simulink model "TestAgeingImpact_Intermediate_CC_Cycles"  (R2024b)
settings: Solver=FixedStepAuto  StartTime=0.0  StopTime=simTime  FixedStep=Ts  RelTol=1e-3
values from neighbouring files (symbols this model uses):
  I_ch = -OneC/Crate*A*p.L_n*p.a_s_n    [TestParallelCells.m]    (also in simu_ageing_Internediaire.m = -OneC/Crate*A_e; simu_ageing_Internediaire_3HYP.m = -OneC/Crate*A_e; simu_effet_ageing.m = -OneC/Crate)
  Ts = p.delta_t    [TestParallelCells.m]    (also in simu_ageing_Internediaire.m; simu_ageing_Internediaire_3HYP.m; simu_effet_ageing.m)
undefined symbols (not defined in the file or in its folder): p
libraries: nesl_utility x9, fl_lib x5, EHMCell_lib x2, BatteryCurrentManagement x1, spspowerguiLib x1
settings Model: Creator=lab01  LastModifiedBy=chloe

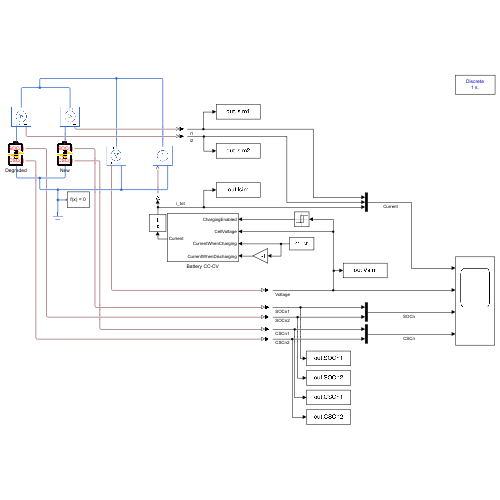
[thumbnail: Simulink's stored preview of the top-level diagram]
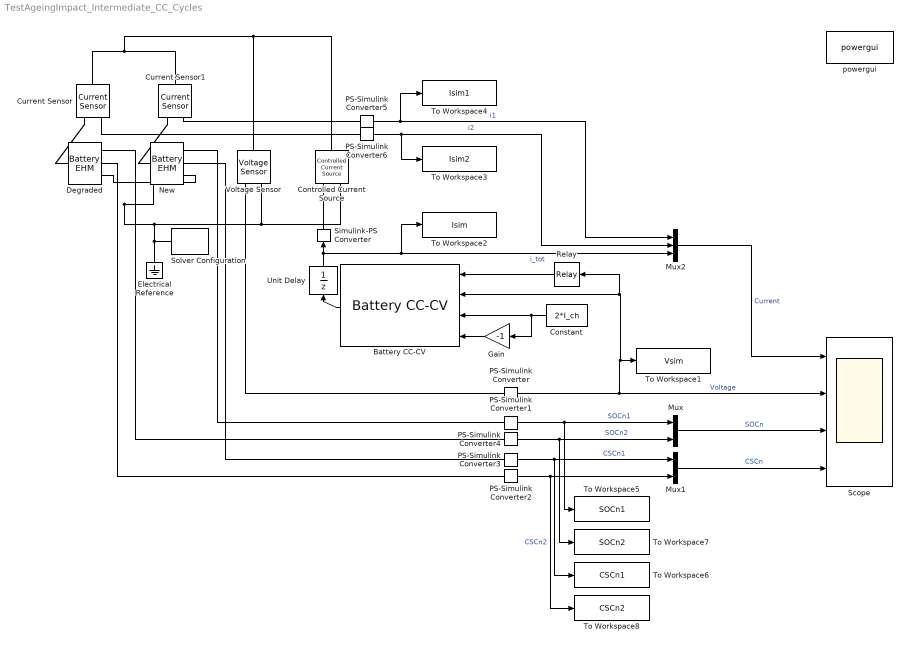
== system TestAgeingImpact_Intermediate_CC_Cycles ==
  Battery CC-CV : BatteryCurrentManagement/Battery CC-CV  MaxCellVoltage=p.volt_max  Kp=100  Ki=10  Kaw=1  Kt=1  Ts=Ts
      settings: LibrarySourceBlock=batt_sl_lib/Current Management/Battery CC-CV
  Constant : Constant  Value=2*I_ch
  Controlled Current Source : fl_lib/Electrical/Electrical Sources/Controlled Current Source
  Current Sensor : fl_lib/Electrical/Electrical Sensors/Current Sensor
  Current Sensor1 : fl_lib/Electrical/Electrical Sensors/Current Sensor
  Degraded : EHMCell_lib/Battery EHM  V0=3.5 V  CI=CI_Inc  epsilon_s_n=p_Inc.epsilon_s_n  epsilon_s_p=p_Inc.epsilon_s_p  n_Li_s=p_Inc.n_Li_s mol  D_s_n0=p_Inc.D_s_n0 m^2/s  R_f_n=p_Inc.R_f_n kg*m^4/(A^2*s^3)  R_f_p=0 kg*m^4/(A^2*s^3)  R_c=0 kg*m^4/(A^2*s^3)
      settings: InternalSimscapePortConfiguration="{\"Bottom\":[{\"id\":\"n\",\"label\":\"-\",\"type\":\"foundation.electrical.electrical\"}],\"Left\":[],\"Right\":[{\"id\":\"SOCn\",\"label\":\"SOC(-)\",\"type\":\"output\"},{\"id\":\"CSCn\",\"label\":\"CSC(-)\",\"type\":\"output\"}],\"Top\":[{\"id\":\"p\",\"label\":\"+\",\"type\":\"foundation.electrical.electrical\"}]}"
  Electrical Reference : fl_lib/Electrical/Electrical Elements/Electrical Reference
  Gain : Gain  Gain=-1
  Mux : Mux  Inputs=2
  Mux1 : Mux  Inputs=2
  Mux2 : Mux  Inputs=3
  New : EHMCell_lib/Battery EHM  V0=3.5 V  CI=0.0235070507454338  epsilon_s_n=0.6  epsilon_s_p=0.5  n_Li_s=2.5 mol  D_s_n0=3.9e-14 m^2/s  R_f_n=1e-3 kg*m^4/(A^2*s^3)  R_f_p=0 kg*m^4/(A^2*s^3)  R_c=0 kg*m^4/(A^2*s^3)
      settings: InternalSimscapePortConfiguration="{\"Bottom\":[{\"id\":\"n\",\"label\":\"-\",\"type\":\"foundation.electrical.electrical\"}],\"Left\":[],\"Right\":[{\"id\":\"SOCn\",\"label\":\"SOC(-)\",\"type\":\"output\"},{\"id\":\"CSCn\",\"label\":\"CSC(-)\",\"type\":\"output\"}],\"Top\":[{\"id\":\"p\",\"label\":\"+\",\"type\":\"foundation.electrical.electrical\"}]}"
  PS-Simulink Converter{,1..6} (7 alike) : nesl_utility/PS-Simulink Converter  PhysicalDomain=network_engine_domain  SubClassName=ps_output  LeftPortType=input  RightPortType=output  PseudoPeriodic=off  Frequencies=[]  VectorFormat=inherit  Unit=inherit  AffineConversion=off
  Relay : Relay  OnSwitchValue=p.volt_max-0.05  OffSwitchValue=p.volt_min+0.05  OnOutputValue=0  OffOutputValue=1
  Scope : Scope  NumInputPorts=4
  Simulink-PS Converter : nesl_utility/Simulink-PS Converter  PhysicalDomain=network_engine_domain  SubClassName=ps_input  LeftPortType=input  RightPortType=output  PseudoPeriodic=off  Frequencies=[]  NoiseDistribution=none  NoiseParameters=[]  Unit=1  AffineConversion=off  FilteringAndDerivatives=provide  SimscapeFilterOrder=1  InputFilterTimeConstant=0.001  UdotUserProvided=0
  Solver Configuration : nesl_utility/Solver Configuration  PhysicalDomain=network_engine_domain  SubClassName=solver  LeftPortType=input  RightPortType=generic  Tones=[]  Harmonics=[]  SimulateNoise=off  Profile=off  UseLocalSampling=off  EnableSwitchedLinearOptims=on  FrequencyDomain=off  UseCCode=off  RelTol=0.001  AbsTol=0.001  MinStep=1e-09  ToWorkspace=off  RevertToSquareIcSolve=off  NumHomotopyIterations=100  PhasorMode=off  PhasorModeNumHarmonics=1  ConsistencySolver=NEWTON_XTOL_AFTER_FTOL  IndexReductionMethod=DerivativeReplacement  DoDC=off  ResidualTolerance=1e-09  ConsistencyTolSource=GLOBAL  ConsistencyAbsTol=0.001  ConsistencyRelTol=0.001  ConsistencyTolFactor=0.001  UseLocalSolver=off  LocalSolverChoice=NE_BACKWARD_EULER_ADVANCER  ResolveIndetEquations=on  FunctionEvalNumThread=1  LocalSolverSampleTime=0.001  DoFixedCost=off  MaxNonlinIter=3  MaxModeIter=2  ComputeImpulses=off  ImpulseIterations=2  LinearAlgebra=auto  LinearAlgebraNumThread=0  EquationFormulation=NE_TIME_EF  DelaysMemoryBudget=1024  AutomaticFiltering=on  FilteringTimeConstant=0.001  PartitionStorageMethod=AS_NEEDED  PartitionMemoryBudget=1024  PartitionMethod=ROBUST  MultibodyUseLocalSolver=off  MultibodyLocalSolverChoice=ODE1  MultibodyLocalSolverSampleTime=0.001
  To Workspace1 : ToWorkspace  VariableName=Vsim  SaveFormat=Timeseries  SampleTime=-1
      settings: Save2DSignal=2-D array (concatenate along first dimension)
  To Workspace2 : ToWorkspace  VariableName=Isim  SaveFormat=Timeseries  SampleTime=-1
      settings: Save2DSignal=2-D array (concatenate along first dimension)
  To Workspace3 : ToWorkspace  VariableName=Isim2  SaveFormat=Timeseries  SampleTime=-1
      settings: Save2DSignal=2-D array (concatenate along first dimension)
  To Workspace4 : ToWorkspace  VariableName=Isim1  SaveFormat=Timeseries  SampleTime=-1
      settings: Save2DSignal=2-D array (concatenate along first dimension)
  To Workspace5 : ToWorkspace  VariableName=SOCn1  SaveFormat=Timeseries  SampleTime=-1
      settings: Save2DSignal=2-D array (concatenate along first dimension)
  To Workspace6 : ToWorkspace  VariableName=CSCn1  SaveFormat=Timeseries  SampleTime=-1
      settings: Save2DSignal=2-D array (concatenate along first dimension)
  To Workspace7 : ToWorkspace  VariableName=SOCn2  SaveFormat=Timeseries  SampleTime=-1
      settings: Save2DSignal=2-D array (concatenate along first dimension)
  To Workspace8 : ToWorkspace  VariableName=CSCn2  SaveFormat=Timeseries  SampleTime=-1
      settings: Save2DSignal=2-D array (concatenate along first dimension)
  Unit Delay : UnitDelay  SampleTime=-1  HasFrameUpgradeWarning=on
  Voltage Sensor : fl_lib/Electrical/Electrical Sensors/Voltage Sensor
  powergui : spspowerguiLib/powergui  Priority=1  SimulationMode=Discrete  SampleTime=Ts  frequency=60  Iterations=50  frequencyindice=60  Pbase=100e6  ErrMax=1e-4  UnitsV=kV  UnitsW=MW  buscounter=0  FunctionMessages=off  echomessages=off  EnableUseOfTLC=off  CurrentSourceSwitches=off  DisableSnubberDevices=off  DisableRonSwitches=off  DisableVfSwitches=off  DisplayEquations=off  AutomaticDiscreteSolvers=off  SolverType=Tustin/Backward Euler (TBE)  Interpol=off  ExternalGateDelay=off  methode=off  Ts=100  x0status=blocks  SPID=on  SwTol=0  HookPort=off  NonlinearTolerance=1e-4  nMaxIteration=100  ContinueOnMaxIteration=off  RestoreLinks=warning  ResistiveCurrentMeasurement=off  Frange=[0:2:500]  Ylog=off  Xlog=on  ShowGrid=off  save=off  variable=ZData  structure=0  ZoomFFT=off  StartTime=0.0  cycles=1  DisplayStyle=1  fundamental=60  FreqAxis=off  MaxFrequency=1000  frequencyindicesteady=1  RmsSteady=1  display=off
  wires:
  PS-Simulink Converter3/1 -> To Workspace6/1, Mux1/1  "CSCn1"
  PS-Simulink Converter2/1 -> To Workspace8/1, Mux1/2  "CSCn2"
  Mux1/1 -> Scope/4  "CSCn"
  Mux/1 -> Scope/3  "SOCn"
  PS-Simulink Converter6/1 -> To Workspace3/1, Mux2/2  "i2"
  PS-Simulink Converter1/1 -> To Workspace5/1, Mux/1  "SOCn1"
  Gain/1 -> Battery CC-CV/4
  Constant/1 -> Gain/1, Battery CC-CV/3
  Unit Delay/1 -> To Workspace2/1, Mux2/3, Simulink-PS Converter/1  "i_tot"
  Battery CC-CV/1 -> Unit Delay/1
  PS-Simulink Converter4/1 -> To Workspace7/1, Mux/2  "SOCn2"
  PS-Simulink Converter/1 -> Relay/1, Battery CC-CV/2, To Workspace1/1, Scope/2  "Voltage"
  Relay/1 -> Battery CC-CV/1
  Mux2/1 -> Scope/1  "Current"
  PS-Simulink Converter5/1 -> To Workspace4/1, Mux2/1  "i1"
  connections:
  Controlled Current Source/RConn2 -- Voltage Sensor/RConn2 -- Solver Configuration/RConn1 -- Electrical Reference/LConn1 -- New/RConn3 -- Degraded/RConn3
  Controlled Current Source/LConn1 -- Voltage Sensor/LConn1 -- Current Sensor/LConn1 -- Current Sensor1/LConn1
  PS-Simulink Converter6/LConn1 -- Current Sensor/RConn1
  PS-Simulink Converter/LConn1 -- Voltage Sensor/RConn1
  Degraded/RConn2 -- PS-Simulink Converter2/LConn1
  New/RConn1 -- PS-Simulink Converter1/LConn1
  Degraded/LConn1 -- Current Sensor/RConn2
  Simulink-PS Converter/RConn1 -- Controlled Current Source/RConn1
  New/RConn2 -- PS-Simulink Converter3/LConn1
  PS-Simulink Converter5/LConn1 -- Current Sensor1/RConn1
  New/LConn1 -- Current Sensor1/RConn2
  Degraded/RConn1 -- PS-Simulink Converter4/LConn1
